simulink model "full_maneuver_platoon_new_strategy"  (R2019a)
settings: Solver=VariableStepAuto  StartTime=0.0  StopTime=70  FixedStep=0.1  MaxStep=0.05  RelTol=1e-3
libraries: simulink x97, dspsigops x7, powerlib_meascontrol x7, autolibshared x7
(part 5 of 7)

== system full_maneuver_platoon_new_strategy/Fo/Regular Vehicle Following/Velocity Control ==
  velocity : Inport
  realInput : Inport  Port=2
  intReset : Inport  Port=3
  Anti-windup gain : Gain  Gain=velKp/velKi
  Integrator2 : Integrator  ExternalReset=falling
  Sum : Sum  Inputs=|+-
  Sum1 : Sum  Inputs=|-+
  Sum2 : Sum  Inputs=-+|
  Sum3 : Sum  Inputs=|++
  freeFlowVel : Constant  Value=freeFlowVel
  velKi : Gain  Gain=velKi
  velKp : Gain  Gain=velKp
  u : Outport
  wires:
  Sum/1 -> velKi/1, velKp/1
  velKp/1 -> Sum3/2
  velKi/1 -> Sum2/2
  Integrator2/1 -> Sum3/1
  velocity/1 -> Sum/2
  freeFlowVel/1 -> Sum/1
  intReset/1 -> Integrator2/2
  Sum3/1 -> Sum1/2, u/1
  Anti-windup gain/1 -> Sum2/1
  realInput/1 -> Sum1/1
  Sum1/1 -> Anti-windup gain/1
  Sum2/1 -> Integrator2/1

== system full_maneuver_platoon_new_strategy/Fo/Vehicle Following During LC/Compute Errors ==
  xf : Inport
  vf : Inport  Port=2
  xl : Inport  Port=3
  vl : Inport  Port=4
  lcFlag : Inport  Port=5
  Compare To Constant : simulink/Logic and Bit Operations/Compare To Constant  relop=<=  const=0  OutDataTypeStr=boolean
  Demux : Demux  Outputs=2
  Demux1 : Demux  Outputs=2
  Gain3 : Gain  Gain=velFilterGain
  Integrator : Integrator  InitialCondition=[h d0]
  Integrator1 : Integrator  InitialCondition=vx0
  Multiply : Product
  Mux : Mux  Inputs=2
  Mux1 : Mux  Inputs=2
  Product : Product
  Saturation : Saturate  UpperLimit=maxAcceleration  LowerLimit=minAcceleration
  Sum : Sum  Inputs=-+|
  Sum1 : Sum  Inputs=++|
  Sum2 : Sum  Inputs=+-|
  Sum3 : Sum  Inputs=|++
  Sum4 : Sum  Inputs=-+|
  Sum5 : Sum  Inputs=|+-
  Sum6 : Sum  Inputs=+-|
  Sum7 : Sum  Inputs=|++
  Sum8 : Sum  Inputs=|+-
  Switch : Switch  Criteria=u2 > Threshold
  d0 : Constant  Value=d0
  d0Lc : Constant  Value=d0Lc
  h : Constant  Value=h
  hFilterGain : Gain  Gain=hFilterGain
  hLc : Constant  Value=hLc
  vLen : Constant  Value=lr+lf
  eh : Outport
  ev : Outport  Port=2
  "gap " : Outport  Port=3
  unsafeFlag : Outport  Port=4
  wires:
  Sum4/1 -> ev/1
  d0Lc/1 -> Mux1/2
  hFilterGain/1 -> Integrator/1
  Demux/1 -> Multiply/2
  xf/1 -> Sum1/2
  Sum/1 -> Sum2/1, "gap "/1, Sum6/1  "gap"
  Multiply/1 -> Sum3/1
  Demux1/2 -> Sum7/2
  hLc/1 -> Mux1/1
  vLen/1 -> Sum1/1
  Demux/2 -> Sum3/2
  Switch/1 -> Sum5/1
  Sum5/1 -> hFilterGain/1
  vf/1 -> Multiply/1, Product/1, Sum4/1
  Sum1/1 -> Sum/1  "x (front bumber)"
  Sum3/1 -> Sum2/2  "desired  gap"
  h/1 -> Mux/1
  Product/1 -> Sum7/1
  xl/1 -> Sum/2
  lcFlag/1 -> Switch/2
  Sum2/1 -> eh/1
  Compare To Constant/1 -> unsafeFlag/1
  Demux1/1 -> Product/2
  Integrator/1 -> Sum5/2, Demux/1
  d0/1 -> Mux/2
  Mux1/1 -> Switch/1
  Sum7/1 -> Sum6/2  "safe  gap"
  Mux/1 -> Switch/3, Demux1/1  "min safe gap"
  Sum6/1 -> Compare To Constant/1
  Saturation/1 -> Integrator1/1
  Gain3/1 -> Saturation/1
  Integrator1/1 -> Sum4/2, Sum8/2
  Sum8/1 -> Gain3/1
  vl/1 -> Sum8/1

== system full_maneuver_platoon_new_strategy/Fo/Vehicle Following During LC/Subsystem ==
  note: Condition for Lane Changing Vehicle
  note: Condition for Gap Generating Vehicle
  ego : Inport  OutDataTypeStr=Bus: vehStatesBus
  futureLeader : Inport  Port=2  OutDataTypeStr=Bus: vehStatesBus
  lcFlag : Inport  Port=3
  AND : Logic  IconShape=distinctive  AllPortsSameDT=off  OutDataTypeStr=boolean
  AND1 : Logic  IconShape=distinctive  AllPortsSameDT=off  OutDataTypeStr=boolean
  Abs : Abs
  Abs1 : Abs
  Bus Selector1 : BusSelector  OutputSignals=Y
  Bus Selector2 : BusSelector  OutputSignals=Y
  Compare To Constant : simulink/Logic and Bit Operations/Compare To Constant  relop=<=  const=1.8  OutDataTypeStr=boolean
  Compare To Constant1 : simulink/Logic and Bit Operations/Compare To Constant  relop=<=  const=0.5  OutDataTypeStr=boolean
  NOT : Logic  Operator=NOT  IconShape=distinctive  AllPortsSameDT=off  OutDataTypeStr=boolean
  OR : Logic  Operator=OR  IconShape=distinctive  AllPortsSameDT=off  OutDataTypeStr=boolean
  Scope : Scope  NumInputPorts=2
  Sum : Sum  Inputs=|+-
  Sum1 : Sum  Inputs=-+|
  lcDone : Outport
  wires:
  futureLeader/1 -> Bus Selector1/1
  Bus Selector1/1 -> Sum1/1, Sum/2  "<Y>"
  AND/1 -> Scope/1, OR/1
  Sum/1 -> Abs1/1
  Compare To Constant/1 -> AND/1
  lcFlag/1 -> AND1/1, NOT/1
  ego/1 -> Bus Selector2/1
  NOT/1 -> AND/2
  Sum1/1 -> Abs/1
  Compare To Constant1/1 -> AND1/2
  OR/1 -> lcDone/1
  AND1/1 -> Scope/2, OR/2
  Bus Selector2/1 -> Sum/1, Sum1/2  "<Y>"
  Abs/1 -> Compare To Constant1/1
  Abs1/1 -> Compare To Constant/1

== system full_maneuver_platoon_new_strategy/Fo/Vehicle Following During LC/Veh Following ==
  eh : Inport
  ev : Inport  Port=2
  realInput : Inport  Port=3
  intReset : Inport  Port=4
  Anti-windup gain : Gain  Gain=sqrt(Ki/Kd)
  Integrator : Integrator  ExternalReset=rising
  Kd : Gain  Gain=Kd
  Ki : Gain  Gain=Ki
  Kp : Gain  Gain=Kp
  Saturation1 : Saturate  UpperLimit=maxHeadwayError  LowerLimit=minHeadwayError
  Scope : Scope  NumInputPorts=4
  Sum : Sum  Inputs=|-+
  Sum1 : Sum  Inputs=+++
  Sum5 : Sum  Inputs=-+|
  u : Outport
  wires:
  intReset/1 -> Integrator/2
  Sum/1 -> Anti-windup gain/1
  realInput/1 -> Sum/1
  Sum1/1 -> Scope/4, u/1, Sum/2
  eh/1 -> Saturation1/1
  Saturation1/1 -> Ki/1, Kp/1
  Kd/1 -> Sum1/3, Scope/3
  Kp/1 -> Scope/2, Sum1/2
  Integrator/1 -> Scope/1, Sum1/1
  Sum5/1 -> Integrator/1
  Anti-windup gain/1 -> Sum5/1
  Ki/1 -> Sum5/2
  ev/1 -> Kd/1

== system full_maneuver_platoon_new_strategy/Fo/Vehicle Following During LC/Velocity Control ==
  velocity : Inport
  realInput : Inport  Port=2
  intReset : Inport  Port=3
  Anti-windup gain : Gain  Gain=velKp/velKi
  Integrator2 : Integrator  ExternalReset=falling
  Sum : Sum  Inputs=|+-
  Sum1 : Sum  Inputs=|-+
  Sum2 : Sum  Inputs=-+|
  Sum3 : Sum  Inputs=|++
  freeFlowVel : Constant  Value=freeFlowVel
  velKi : Gain  Gain=velKi
  velKp : Gain  Gain=velKp
  u : Outport
  wires:
  Sum2/1 -> Integrator2/1
  Sum1/1 -> Anti-windup gain/1
  realInput/1 -> Sum1/1
  Anti-windup gain/1 -> Sum2/1
  Sum3/1 -> u/1, Sum1/2
  intReset/1 -> Integrator2/2
  freeFlowVel/1 -> Sum/1
  velocity/1 -> Sum/2
  Integrator2/1 -> Sum3/1
  velKi/1 -> Sum2/2
  velKp/1 -> Sum3/2
  Sum/1 -> velKp/1, velKi/1

== system full_maneuver_platoon_new_strategy/Fo/Virtual Vehicle Following/Compute Errors ==
  xf : Inport
  vf : Inport  Port=2
  xl : Inport  Port=3
  vl : Inport  Port=4
  lcFlag : Inport  Port=5
  Compare To Constant : simulink/Logic and Bit Operations/Compare To Constant  relop=<=  const=0  OutDataTypeStr=boolean
  Demux : Demux  Outputs=2
  Demux1 : Demux  Outputs=2
  Gain3 : Gain  Gain=velFilterGain/10
  Integrator : Integrator  InitialCondition=[h d0]
  Integrator1 : Integrator  InitialCondition=vx0
  Multiply : Product
  Mux : Mux  Inputs=2
  Mux1 : Mux  Inputs=2
  Product : Product
  Saturation : Saturate  UpperLimit=maxAcceleration  LowerLimit=minAcceleration
  Sum : Sum  Inputs=-+|
  Sum1 : Sum  Inputs=++|
  Sum2 : Sum  Inputs=+-|
  Sum3 : Sum  Inputs=|++
  Sum4 : Sum  Inputs=-+|
  Sum5 : Sum  Inputs=|+-
  Sum6 : Sum  Inputs=+-|
  Sum7 : Sum  Inputs=|++
  Sum8 : Sum  Inputs=|+-
  Switch : Switch  Criteria=u2 > Threshold
  d0 : Constant  Value=d0
  d0Lc : Constant  Value=d0Lc
  h : Constant  Value=h
  hFilterGain : Gain  Gain=hFilterGain
  hLc : Constant  Value=hLc
  vLen : Constant  Value=lr+lf
  eh : Outport
  ev : Outport  Port=2
  "gap " : Outport  Port=3
  unsafeFlag : Outport  Port=4
  wires:
  Sum6/1 -> Compare To Constant/1
  Mux/1 -> Demux1/1, Switch/3  "min safe gap"
  Sum7/1 -> Sum6/2  "safe  gap"
  Mux1/1 -> Switch/1
  d0/1 -> Mux/2
  Integrator/1 -> Demux/1, Sum5/2
  Demux1/1 -> Product/2
  Compare To Constant/1 -> unsafeFlag/1
  Sum2/1 -> eh/1
  lcFlag/1 -> Switch/2
  xl/1 -> Sum/2
  Product/1 -> Sum7/1
  h/1 -> Mux/1
  Sum3/1 -> Sum2/2  "desired  gap"
  Sum1/1 -> Sum/1  "x (front bumber)"
  vf/1 -> Sum4/1, Product/1, Multiply/1
  Sum5/1 -> hFilterGain/1
  Switch/1 -> Sum5/1
  Demux/2 -> Sum3/2
  vLen/1 -> Sum1/1
  hLc/1 -> Mux1/1
  Demux1/2 -> Sum7/2
  Multiply/1 -> Sum3/1
  Sum/1 -> Sum6/1, "gap "/1, Sum2/1  "gap"
  xf/1 -> Sum1/2
  Demux/1 -> Multiply/2
  hFilterGain/1 -> Integrator/1
  d0Lc/1 -> Mux1/2
  Sum4/1 -> ev/1
  Integrator1/1 -> Sum4/2, Sum8/2
  Gain3/1 -> Saturation/1
  Sum8/1 -> Gain3/1
  Saturation/1 -> Integrator1/1
  vl/1 -> Sum8/1

== system full_maneuver_platoon_new_strategy/Fo/Virtual Vehicle Following/Subsystem ==
  ego : Inport  OutDataTypeStr=Bus: vehStatesBus
  virtualLeader : Inport  Port=2  OutDataTypeStr=Bus: vehStatesBus
  Abs : Abs
  Bus Selector : BusSelector  OutputSignals=Y
  Bus Selector1 : BusSelector  OutputSignals=Y
  Compare To Constant : simulink/Logic and Bit Operations/Compare To Constant  relop=<  const=3.6-0.5  OutDataTypeStr=boolean
  Scope : Scope  NumInputPorts=3
  Sum : Sum  Inputs=+-
  lcStarted : Outport
  wires:
  ego/1 -> Bus Selector/1
  virtualLeader/1 -> Bus Selector1/1
  Bus Selector/1 -> Scope/1, Sum/1  "<Y>"
  Bus Selector1/1 -> Sum/2, Scope/2  "<Y>"
  Compare To Constant/1 -> lcStarted/1
  Sum/1 -> Abs/1
  Abs/1 -> Scope/3, Compare To Constant/1

== system full_maneuver_platoon_new_strategy/Fo/Virtual Vehicle Following/Velocity Control ==
  note: Velocity control
  intReset : Inport
  ev : Inport  Port=2
  Integrator2 : Integrator  ExternalReset=rising
  Sum3 : Sum
  velKi : Gain  Gain=velKi
  velKp : Gain  Gain=velKp
  Out1 : Outport
  wires:
  Integrator2/1 -> velKi/1
  velKi/1 -> Sum3/2
  Sum3/1 -> Out1/1
  velKp/1 -> Sum3/1
  ev/1 -> velKp/1, Integrator2/1
  intReset/1 -> Integrator2/2

== system full_maneuver_platoon_new_strategy/Fo/Virtual Vehicle Following/Virtual Leader Following ==
  eh : Inport
  ev : Inport  Port=2
  realInput : Inport  Port=3
  Anti-windup gain : Gain  Gain=sqrt(Ki/Kd)
  Integrator : Integrator
  Kd : Gain  Gain=Kd
  Ki : Gain  Gain=Ki
  Kp : Gain  Gain=Kp
  Saturation1 : Saturate  UpperLimit=maxHeadwayError  LowerLimit=minHeadwayError
  Scope : Scope  NumInputPorts=3
  Sum : Sum  Inputs=|-+
  Sum1 : Sum  Inputs=+++
  Sum5 : Sum  Inputs=-+|
  u : Outport
  wires:
  ev/1 -> Kd/1
  Ki/1 -> Sum5/2
  Anti-windup gain/1 -> Sum5/1
  Sum5/1 -> Integrator/1
  Integrator/1 -> Scope/1, Sum1/1
  Kp/1 -> Scope/2, Sum1/2
  Kd/1 -> Scope/3, Sum1/3
  Saturation1/1 -> Kp/1, Ki/1
  eh/1 -> Saturation1/1
  Sum1/1 -> Sum/2, u/1
  realInput/1 -> Sum/1
  Sum/1 -> Anti-windup gain/1

== system full_maneuver_platoon_new_strategy/Fo/followerErrors/gapToFollower ==
  xf : Inport
  vf : Inport  Port=2
  xl : Inport  Port=3
  Multiply : Product
  Sum : Sum  Inputs=-+|
  Sum1 : Sum  Inputs=++|
  Sum2 : Sum  Inputs=+-|
  Sum3 : Sum  Inputs=|++
  d0 : Constant  Value=d0
  h : Constant  Value=h
  vLen : Constant  Value=lr+lf
  eh : Outport
  "gap " : Outport  Port=2
  wires:
  vLen/1 -> Sum1/1
  Multiply/1 -> Sum3/1
  Sum/1 -> "gap "/1, Sum2/1  "gap"
  xf/1 -> Sum1/2
  Sum3/1 -> Sum2/2  "desired  gap"
  vf/1 -> Multiply/1
  Sum1/1 -> Sum/1  "x (front bumber)"
  xl/1 -> Sum/2
  Sum2/1 -> eh/1
  h/1 -> Multiply/2  "time headway"
  d0/1 -> Sum3/2  "gap at  standstill"

== system full_maneuver_platoon_new_strategy/Ld/Lateral Control/Full State Observer ==
  note: yhat
  note: xhat
  measuredOutputs : Inport
  delta : Inport  Port=2
  Add1 : Sum  Inputs=|-+
  Gain : Gain  Gain=B  Multiplication=Matrix(K*u)
  Gain1 : Gain  Gain=C  Multiplication=Matrix(K*u)
  Gain2 : Gain  Gain=L  Multiplication=Matrix(K*u)
  Gain3 : Gain  Gain=A  Multiplication=Matrix(K*u)
  Integrator : Integrator  InitialCondition=[y0; 0; 0; 0]
  Signal Specification : SignalSpecification  Dimensions=[size(C,1) 1]
  Sum : Sum  Inputs=+++
  xhat : Outport
  wires:
  Gain2/1 -> Sum/1
  Signal Specification/1 -> Gain2/1
  Gain3/1 -> Sum/2
  Gain/1 -> Sum/3
  delta/1 -> Gain/1
  measuredOutputs/1 -> Add1/2
  Sum/1 -> Integrator/1
  Gain1/1 -> Add1/1
  Integrator/1 -> Gain1/1, Gain3/1, xhat/1
  Add1/1 -> Signal Specification/1

== system full_maneuver_platoon_new_strategy/Ld/Lateral Control/Triggered Subsystem1 ==
  In1 : Inport
  Trigger : TriggerPort  VariantControl=Variant
  Out1 : Outport  InitialOutput=y0
  wires:
  In1/1 -> Out1/1

== system full_maneuver_platoon_new_strategy/Ld/Regular Vehicle Following/Compute Errors ==
  xf : Inport
  vf : Inport  Port=2
  xl : Inport  Port=3
  vl : Inport  Port=4
  lcFlag : Inport  Port=5
  Compare To Constant : simulink/Logic and Bit Operations/Compare To Constant  relop=<=  const=0  OutDataTypeStr=boolean
  Demux : Demux  Outputs=2
  Demux1 : Demux  Outputs=2
  Gain3 : Gain  Gain=velFilterGain
  Integrator : Integrator  InitialCondition=[h d0]
  Integrator1 : Integrator  InitialCondition=vx0
  Multiply : Product
  Mux : Mux  Inputs=2
  Mux1 : Mux  Inputs=2
  Product : Product
  Saturation : Saturate  UpperLimit=maxAcceleration  LowerLimit=minAcceleration
  Sum : Sum  Inputs=-+|
  Sum1 : Sum  Inputs=++|
  Sum2 : Sum  Inputs=+-|
  Sum3 : Sum  Inputs=|++
  Sum4 : Sum  Inputs=-+|
  Sum5 : Sum  Inputs=|+-
  Sum6 : Sum  Inputs=+-|
  Sum7 : Sum  Inputs=|++
  Sum8 : Sum  Inputs=|+-
  Switch : Switch  Criteria=u2 > Threshold
  d0 : Constant  Value=d0
  d0Lc : Constant  Value=d0Lc
  h : Constant  Value=h
  hFilterGain : Gain  Gain=hFilterGain
  hLc : Constant  Value=hLc
  vLen : Constant  Value=lr+lf
  eh : Outport
  ev : Outport  Port=2
  "gap " : Outport  Port=3
  unsafeFlag : Outport  Port=4
  wires:
  Sum6/1 -> Compare To Constant/1
  Mux/1 -> Demux1/1, Switch/3  "min safe gap"
  Sum7/1 -> Sum6/2  "safe  gap"
  Mux1/1 -> Switch/1
  d0/1 -> Mux/2
  Integrator/1 -> Demux/1, Sum5/2
  Demux1/1 -> Product/2
  Compare To Constant/1 -> unsafeFlag/1
  Sum2/1 -> eh/1
  lcFlag/1 -> Switch/2
  xl/1 -> Sum/2
  Product/1 -> Sum7/1
  h/1 -> Mux/1
  Sum3/1 -> Sum2/2  "desired  gap"
  Sum1/1 -> Sum/1  "x (front bumber)"
  vf/1 -> Sum4/1, Product/1, Multiply/1
  Sum5/1 -> hFilterGain/1
  Switch/1 -> Sum5/1
  Demux/2 -> Sum3/2
  vLen/1 -> Sum1/1
  hLc/1 -> Mux1/1
  Demux1/2 -> Sum7/2
  Multiply/1 -> Sum3/1
  Sum/1 -> Sum6/1, "gap "/1, Sum2/1  "gap"
  xf/1 -> Sum1/2
  Demux/1 -> Multiply/2
  hFilterGain/1 -> Integrator/1
  d0Lc/1 -> Mux1/2
  vl/1 -> Sum8/1
  Sum4/1 -> ev/1
  Gain3/1 -> Saturation/1
  Saturation/1 -> Integrator1/1
  Integrator1/1 -> Sum4/2, Sum8/2
  Sum8/1 -> Gain3/1

== system full_maneuver_platoon_new_strategy/Ld/Regular Vehicle Following/Veh Following ==
  eh : Inport
  ev : Inport  Port=2
  realInput : Inport  Port=3
  intReset : Inport  Port=4
  Anti-windup gain : Gain  Gain=sqrt(Ki/Kd)
  Integrator : Integrator  ExternalReset=rising
  Kd : Gain  Gain=Kd
  Ki : Gain  Gain=Ki
  Kp : Gain  Gain=Kp
  Saturation1 : Saturate  UpperLimit=maxHeadwayError  LowerLimit=minHeadwayError
  Scope : Scope  NumInputPorts=4
  Sum : Sum  Inputs=|-+
  Sum1 : Sum  Inputs=+++
  Sum5 : Sum  Inputs=-+|
  u : Outport
  wires:
  ev/1 -> Kd/1
  Ki/1 -> Sum5/2
  Anti-windup gain/1 -> Sum5/1
  Sum5/1 -> Integrator/1
  Integrator/1 -> Sum1/1, Scope/1
  Kp/1 -> Sum1/2, Scope/2
  Kd/1 -> Scope/3, Sum1/3
  Saturation1/1 -> Kp/1, Ki/1
  eh/1 -> Saturation1/1
  Sum1/1 -> Sum/2, u/1, Scope/4
  realInput/1 -> Sum/1
  Sum/1 -> Anti-windup gain/1
  intReset/1 -> Integrator/2

== system full_maneuver_platoon_new_strategy/Ld/Regular Vehicle Following/Velocity Control ==
  velocity : Inport
  realInput : Inport  Port=2
  intReset : Inport  Port=3
  Anti-windup gain : Gain  Gain=velKp/velKi
  Integrator2 : Integrator  ExternalReset=falling
  Sum : Sum  Inputs=|+-
  Sum1 : Sum  Inputs=|-+
  Sum2 : Sum  Inputs=-+|
  Sum3 : Sum  Inputs=|++
  freeFlowVel : Constant  Value=freeFlowVel
  velKi : Gain  Gain=velKi
  velKp : Gain  Gain=velKp
  u : Outport
  wires:
  Sum/1 -> velKi/1, velKp/1
  velKp/1 -> Sum3/2
  velKi/1 -> Sum2/2
  Integrator2/1 -> Sum3/1
  velocity/1 -> Sum/2
  freeFlowVel/1 -> Sum/1
  intReset/1 -> Integrator2/2
  Sum3/1 -> Sum1/2, u/1
  Anti-windup gain/1 -> Sum2/1
  realInput/1 -> Sum1/1
  Sum1/1 -> Anti-windup gain/1
  Sum2/1 -> Integrator2/1

== system full_maneuver_platoon_new_strategy/Ld/Vehicle Following During LC/Compute Errors ==
  xf : Inport
  vf : Inport  Port=2
  xl : Inport  Port=3
  vl : Inport  Port=4
  lcFlag : Inport  Port=5
  Compare To Constant : simulink/Logic and Bit Operations/Compare To Constant  relop=<=  const=0  OutDataTypeStr=boolean
  Demux : Demux  Outputs=2
  Demux1 : Demux  Outputs=2
  Gain3 : Gain  Gain=velFilterGain
  Integrator : Integrator  InitialCondition=[h d0]
  Integrator1 : Integrator  InitialCondition=vx0
  Multiply : Product
  Mux : Mux  Inputs=2
  Mux1 : Mux  Inputs=2
  Product : Product
  Saturation : Saturate  UpperLimit=maxAcceleration  LowerLimit=minAcceleration
  Sum : Sum  Inputs=-+|
  Sum1 : Sum  Inputs=++|
  Sum2 : Sum  Inputs=+-|
  Sum3 : Sum  Inputs=|++
  Sum4 : Sum  Inputs=-+|
  Sum5 : Sum  Inputs=|+-
  Sum6 : Sum  Inputs=+-|
  Sum7 : Sum  Inputs=|++
  Sum8 : Sum  Inputs=|+-
  Switch : Switch  Criteria=u2 > Threshold
  d0 : Constant  Value=d0
  d0Lc : Constant  Value=d0Lc
  h : Constant  Value=h
  hFilterGain : Gain  Gain=hFilterGain
  hLc : Constant  Value=hLc
  vLen : Constant  Value=lr+lf
  eh : Outport
  ev : Outport  Port=2
  "gap " : Outport  Port=3
  unsafeFlag : Outport  Port=4
  wires:
  Sum4/1 -> ev/1
  d0Lc/1 -> Mux1/2
  hFilterGain/1 -> Integrator/1
  Demux/1 -> Multiply/2
  xf/1 -> Sum1/2
  Sum/1 -> Sum2/1, "gap "/1, Sum6/1  "gap"
  Multiply/1 -> Sum3/1
  Demux1/2 -> Sum7/2
  hLc/1 -> Mux1/1
  vLen/1 -> Sum1/1
  Demux/2 -> Sum3/2
  Switch/1 -> Sum5/1
  Sum5/1 -> hFilterGain/1
  vf/1 -> Multiply/1, Product/1, Sum4/1
  Sum1/1 -> Sum/1  "x (front bumber)"
  Sum3/1 -> Sum2/2  "desired  gap"
  h/1 -> Mux/1
  Product/1 -> Sum7/1
  xl/1 -> Sum/2
  lcFlag/1 -> Switch/2
  Sum2/1 -> eh/1
  Compare To Constant/1 -> unsafeFlag/1
  Demux1/1 -> Product/2
  Integrator/1 -> Sum5/2, Demux/1
  d0/1 -> Mux/2
  Mux1/1 -> Switch/1
  Sum7/1 -> Sum6/2  "safe  gap"
  Mux/1 -> Switch/3, Demux1/1  "min safe gap"
  Sum6/1 -> Compare To Constant/1
  Saturation/1 -> Integrator1/1
  Gain3/1 -> Saturation/1
  Integrator1/1 -> Sum4/2, Sum8/2
  Sum8/1 -> Gain3/1
  vl/1 -> Sum8/1

== system full_maneuver_platoon_new_strategy/Ld/Vehicle Following During LC/Subsystem ==
  note: Condition for Lane Changing Vehicle
  note: Condition for Gap Generating Vehicle
  ego : Inport  OutDataTypeStr=Bus: vehStatesBus
  futureLeader : Inport  Port=2  OutDataTypeStr=Bus: vehStatesBus
  lcFlag : Inport  Port=3
  AND : Logic  IconShape=distinctive  AllPortsSameDT=off  OutDataTypeStr=boolean
  AND1 : Logic  IconShape=distinctive  AllPortsSameDT=off  OutDataTypeStr=boolean
  Abs : Abs
  Abs1 : Abs
  Bus Selector1 : BusSelector  OutputSignals=Y
  Bus Selector2 : BusSelector  OutputSignals=Y
  Compare To Constant : simulink/Logic and Bit Operations/Compare To Constant  relop=<=  const=1.8  OutDataTypeStr=boolean
  Compare To Constant1 : simulink/Logic and Bit Operations/Compare To Constant  relop=<=  const=0.5  OutDataTypeStr=boolean
  NOT : Logic  Operator=NOT  IconShape=distinctive  AllPortsSameDT=off  OutDataTypeStr=boolean
  OR : Logic  Operator=OR  IconShape=distinctive  AllPortsSameDT=off  OutDataTypeStr=boolean
  Scope : Scope  NumInputPorts=2
  Sum : Sum  Inputs=|+-
  Sum1 : Sum  Inputs=-+|
  lcDone : Outport
  wires:
  futureLeader/1 -> Bus Selector1/1
  Bus Selector1/1 -> Sum1/1, Sum/2  "<Y>"
  AND/1 -> Scope/1, OR/1
  Sum/1 -> Abs1/1
  Compare To Constant/1 -> AND/1
  lcFlag/1 -> AND1/1, NOT/1
  ego/1 -> Bus Selector2/1
  NOT/1 -> AND/2
  Sum1/1 -> Abs/1
  Compare To Constant1/1 -> AND1/2
  OR/1 -> lcDone/1
  AND1/1 -> Scope/2, OR/2
  Bus Selector2/1 -> Sum/1, Sum1/2  "<Y>"
  Abs/1 -> Compare To Constant1/1
  Abs1/1 -> Compare To Constant/1

== system full_maneuver_platoon_new_strategy/Ld/Vehicle Following During LC/Veh Following ==
  eh : Inport
  ev : Inport  Port=2
  realInput : Inport  Port=3
  intReset : Inport  Port=4
  Anti-windup gain : Gain  Gain=sqrt(Ki/Kd)
  Integrator : Integrator  ExternalReset=rising
  Kd : Gain  Gain=Kd
  Ki : Gain  Gain=Ki
  Kp : Gain  Gain=Kp
  Saturation1 : Saturate  UpperLimit=maxHeadwayError  LowerLimit=minHeadwayError
  Scope : Scope  NumInputPorts=4
  Sum : Sum  Inputs=|-+
  Sum1 : Sum  Inputs=+++
  Sum5 : Sum  Inputs=-+|
  u : Outport
  wires:
  intReset/1 -> Integrator/2
  Sum/1 -> Anti-windup gain/1
  realInput/1 -> Sum/1
  Sum1/1 -> Scope/4, u/1, Sum/2
  eh/1 -> Saturation1/1
  Saturation1/1 -> Ki/1, Kp/1
  Kd/1 -> Sum1/3, Scope/3
  Kp/1 -> Scope/2, Sum1/2
  Integrator/1 -> Scope/1, Sum1/1
  Sum5/1 -> Integrator/1
  Anti-windup gain/1 -> Sum5/1
  Ki/1 -> Sum5/2
  ev/1 -> Kd/1

== system full_maneuver_platoon_new_strategy/Ld/Vehicle Following During LC/Velocity Control ==
  velocity : Inport
  realInput : Inport  Port=2
  intReset : Inport  Port=3
  Anti-windup gain : Gain  Gain=velKp/velKi
  Integrator2 : Integrator  ExternalReset=falling
  Sum : Sum  Inputs=|+-
  Sum1 : Sum  Inputs=|-+
  Sum2 : Sum  Inputs=-+|
  Sum3 : Sum  Inputs=|++
  freeFlowVel : Constant  Value=freeFlowVel
  velKi : Gain  Gain=velKi
  velKp : Gain  Gain=velKp
  u : Outport
  wires:
  Sum2/1 -> Integrator2/1
  Sum1/1 -> Anti-windup gain/1
  realInput/1 -> Sum1/1
  Anti-windup gain/1 -> Sum2/1
  Sum3/1 -> u/1, Sum1/2
  intReset/1 -> Integrator2/2
  freeFlowVel/1 -> Sum/1
  velocity/1 -> Sum/2
  Integrator2/1 -> Sum3/1
  velKi/1 -> Sum2/2
  velKp/1 -> Sum3/2
  Sum/1 -> velKp/1, velKi/1

== system full_maneuver_platoon_new_strategy/Ld/Virtual Vehicle Following/Compute Errors ==
  xf : Inport
  vf : Inport  Port=2
  xl : Inport  Port=3
  vl : Inport  Port=4
  lcFlag : Inport  Port=5
  Compare To Constant : simulink/Logic and Bit Operations/Compare To Constant  relop=<=  const=0  OutDataTypeStr=boolean
  Demux : Demux  Outputs=2
  Demux1 : Demux  Outputs=2
  Gain3 : Gain  Gain=velFilterGain/10
  Integrator : Integrator  InitialCondition=[h d0]
  Integrator1 : Integrator  InitialCondition=vx0
  Multiply : Product
  Mux : Mux  Inputs=2
  Mux1 : Mux  Inputs=2
  Product : Product
  Saturation : Saturate  UpperLimit=maxAcceleration  LowerLimit=minAcceleration
  Sum : Sum  Inputs=-+|
  Sum1 : Sum  Inputs=++|
  Sum2 : Sum  Inputs=+-|
  Sum3 : Sum  Inputs=|++
  Sum4 : Sum  Inputs=-+|
  Sum5 : Sum  Inputs=|+-
  Sum6 : Sum  Inputs=+-|
  Sum7 : Sum  Inputs=|++
  Sum8 : Sum  Inputs=|+-
  Switch : Switch  Criteria=u2 > Threshold
  d0 : Constant  Value=d0
  d0Lc : Constant  Value=d0Lc
  h : Constant  Value=h
  hFilterGain : Gain  Gain=hFilterGain
  hLc : Constant  Value=hLc
  vLen : Constant  Value=lr+lf
  eh : Outport
  ev : Outport  Port=2
  "gap " : Outport  Port=3
  unsafeFlag : Outport  Port=4
  wires:
  Sum6/1 -> Compare To Constant/1
  Mux/1 -> Demux1/1, Switch/3  "min safe gap"
  Sum7/1 -> Sum6/2  "safe  gap"
  Mux1/1 -> Switch/1
  d0/1 -> Mux/2
  Integrator/1 -> Demux/1, Sum5/2
  Demux1/1 -> Product/2
  Compare To Constant/1 -> unsafeFlag/1
  Sum2/1 -> eh/1
  lcFlag/1 -> Switch/2
  xl/1 -> Sum/2
  Product/1 -> Sum7/1
  h/1 -> Mux/1
  Sum3/1 -> Sum2/2  "desired  gap"
  Sum1/1 -> Sum/1  "x (front bumber)"
  vf/1 -> Sum4/1, Product/1, Multiply/1
  Sum5/1 -> hFilterGain/1
  Switch/1 -> Sum5/1
  Demux/2 -> Sum3/2
  vLen/1 -> Sum1/1
  hLc/1 -> Mux1/1
  Demux1/2 -> Sum7/2
  Multiply/1 -> Sum3/1
  Sum/1 -> Sum6/1, "gap "/1, Sum2/1  "gap"
  xf/1 -> Sum1/2
  Demux/1 -> Multiply/2
  hFilterGain/1 -> Integrator/1
  d0Lc/1 -> Mux1/2
  Sum4/1 -> ev/1
  Integrator1/1 -> Sum4/2, Sum8/2
  Gain3/1 -> Saturation/1
  Sum8/1 -> Gain3/1
  Saturation/1 -> Integrator1/1
  vl/1 -> Sum8/1

== system full_maneuver_platoon_new_strategy/Ld/Virtual Vehicle Following/Subsystem ==
  ego : Inport  OutDataTypeStr=Bus: vehStatesBus
  virtualLeader : Inport  Port=2  OutDataTypeStr=Bus: vehStatesBus
  Abs : Abs
  Bus Selector : BusSelector  OutputSignals=Y
  Bus Selector1 : BusSelector  OutputSignals=Y
  Compare To Constant : simulink/Logic and Bit Operations/Compare To Constant  relop=<  const=3.6-0.5  OutDataTypeStr=boolean
  Scope : Scope  NumInputPorts=3
  Sum : Sum  Inputs=+-
  lcStarted : Outport
  wires:
  ego/1 -> Bus Selector/1
  virtualLeader/1 -> Bus Selector1/1
  Bus Selector/1 -> Scope/1, Sum/1  "<Y>"
  Bus Selector1/1 -> Sum/2, Scope/2  "<Y>"
  Compare To Constant/1 -> lcStarted/1
  Sum/1 -> Abs/1
  Abs/1 -> Scope/3, Compare To Constant/1

== system full_maneuver_platoon_new_strategy/Ld/Virtual Vehicle Following/Velocity Control ==
  note: Velocity control
  intReset : Inport
  ev : Inport  Port=2
  Integrator2 : Integrator  ExternalReset=rising
  Sum3 : Sum
  velKi : Gain  Gain=velKi
  velKp : Gain  Gain=velKp
  Out1 : Outport
  wires:
  Integrator2/1 -> velKi/1
  velKi/1 -> Sum3/2
  Sum3/1 -> Out1/1
  velKp/1 -> Sum3/1
  ev/1 -> velKp/1, Integrator2/1
  intReset/1 -> Integrator2/2

== system full_maneuver_platoon_new_strategy/Ld/Virtual Vehicle Following/Virtual Leader Following ==
  eh : Inport
  ev : Inport  Port=2
  realInput : Inport  Port=3
  Anti-windup gain : Gain  Gain=sqrt(Ki/Kd)
  Integrator : Integrator
  Kd : Gain  Gain=Kd
  Ki : Gain  Gain=Ki
  Kp : Gain  Gain=Kp
  Saturation1 : Saturate  UpperLimit=maxHeadwayError  LowerLimit=minHeadwayError
  Scope : Scope  NumInputPorts=3
  Sum : Sum  Inputs=|-+
  Sum1 : Sum  Inputs=+++
  Sum5 : Sum  Inputs=-+|
  u : Outport
  wires:
  ev/1 -> Kd/1
  Ki/1 -> Sum5/2
  Anti-windup gain/1 -> Sum5/1
  Sum5/1 -> Integrator/1
  Integrator/1 -> Scope/1, Sum1/1
  Kp/1 -> Scope/2, Sum1/2
  Kd/1 -> Scope/3, Sum1/3
  Saturation1/1 -> Kp/1, Ki/1
  eh/1 -> Saturation1/1
  Sum1/1 -> Sum/2, u/1
  realInput/1 -> Sum/1
  Sum/1 -> Anti-windup gain/1

== system full_maneuver_platoon_new_strategy/Ld/followerErrors/gapToFollower ==
  xf : Inport
  vf : Inport  Port=2
  xl : Inport  Port=3
  Multiply : Product
  Sum : Sum  Inputs=-+|
  Sum1 : Sum  Inputs=++|
  Sum2 : Sum  Inputs=+-|
  Sum3 : Sum  Inputs=|++
  d0 : Constant  Value=d0
  h : Constant  Value=h
  vLen : Constant  Value=lr+lf
  eh : Outport
  "gap " : Outport  Port=2
  wires:
  vLen/1 -> Sum1/1
  Multiply/1 -> Sum3/1
  Sum/1 -> "gap "/1, Sum2/1  "gap"
  xf/1 -> Sum1/2
  Sum3/1 -> Sum2/2  "desired  gap"
  vf/1 -> Multiply/1
  Sum1/1 -> Sum/1  "x (front bumber)"
  xl/1 -> Sum/2
  Sum2/1 -> eh/1
  h/1 -> Multiply/2  "time headway"
  d0/1 -> Sum3/2  "gap at  standstill"

== system full_maneuver_platoon_new_strategy/Lo/Lateral Control/Full State Observer ==
  note: xhat
  note: yhat
  measuredOutputs : Inport
  delta : Inport  Port=2
  Add1 : Sum  Inputs=|-+
  Gain : Gain  Gain=B  Multiplication=Matrix(K*u)
  Gain1 : Gain  Gain=C  Multiplication=Matrix(K*u)
  Gain2 : Gain  Gain=L  Multiplication=Matrix(K*u)
  Gain3 : Gain  Gain=A  Multiplication=Matrix(K*u)
  Integrator : Integrator  InitialCondition=[y0; 0; 0; 0]
  Signal Specification : SignalSpecification  Dimensions=[size(C,1) 1]
  Sum : Sum  Inputs=+++
  xhat : Outport
  wires:
  Add1/1 -> Signal Specification/1
  Integrator/1 -> xhat/1, Gain3/1, Gain1/1
  Gain1/1 -> Add1/1
  Sum/1 -> Integrator/1
  measuredOutputs/1 -> Add1/2
  delta/1 -> Gain/1
  Gain/1 -> Sum/3
  Gain3/1 -> Sum/2
  Signal Specification/1 -> Gain2/1
  Gain2/1 -> Sum/1

== system full_maneuver_platoon_new_strategy/Lo/Lateral Control/Triggered Subsystem1 ==
  In1 : Inport
  Trigger : TriggerPort  VariantControl=Variant
  Out1 : Outport  InitialOutput=y0
  wires:
  In1/1 -> Out1/1

== system full_maneuver_platoon_new_strategy/Lo/Regular Vehicle Following/Compute Errors ==
  xf : Inport
  vf : Inport  Port=2
  xl : Inport  Port=3
  vl : Inport  Port=4
  lcFlag : Inport  Port=5
  Compare To Constant : simulink/Logic and Bit Operations/Compare To Constant  relop=<=  const=0  OutDataTypeStr=boolean
  Demux : Demux  Outputs=2
  Demux1 : Demux  Outputs=2
  Gain3 : Gain  Gain=velFilterGain
  Integrator : Integrator  InitialCondition=[h d0]
  Integrator1 : Integrator  InitialCondition=vx0
  Multiply : Product
  Mux : Mux  Inputs=2
  Mux1 : Mux  Inputs=2
  Product : Product
  Saturation : Saturate  UpperLimit=maxAcceleration  LowerLimit=minAcceleration
  Sum : Sum  Inputs=-+|
  Sum1 : Sum  Inputs=++|
  Sum2 : Sum  Inputs=+-|
  Sum3 : Sum  Inputs=|++
  Sum4 : Sum  Inputs=-+|
  Sum5 : Sum  Inputs=|+-
  Sum6 : Sum  Inputs=+-|
  Sum7 : Sum  Inputs=|++
  Sum8 : Sum  Inputs=|+-
  Switch : Switch  Criteria=u2 > Threshold
  d0 : Constant  Value=d0
  d0Lc : Constant  Value=d0Lc
  h : Constant  Value=h
  hFilterGain : Gain  Gain=hFilterGain
  hLc : Constant  Value=hLc
  vLen : Constant  Value=lr+lf
  eh : Outport
  ev : Outport  Port=2
  "gap " : Outport  Port=3
  unsafeFlag : Outport  Port=4
  wires:
  Sum8/1 -> Gain3/1
  Integrator1/1 -> Sum8/2, Sum4/2
  Saturation/1 -> Integrator1/1
  Gain3/1 -> Saturation/1
  Sum4/1 -> ev/1
  vl/1 -> Sum8/1
  d0Lc/1 -> Mux1/2
  hFilterGain/1 -> Integrator/1
  Demux/1 -> Multiply/2
  xf/1 -> Sum1/2
  Sum/1 -> Sum2/1, "gap "/1, Sum6/1  "gap"
  Multiply/1 -> Sum3/1
  Demux1/2 -> Sum7/2
  hLc/1 -> Mux1/1
  vLen/1 -> Sum1/1
  Demux/2 -> Sum3/2
  Switch/1 -> Sum5/1
  Sum5/1 -> hFilterGain/1
  vf/1 -> Multiply/1, Product/1, Sum4/1
  Sum1/1 -> Sum/1  "x (front bumber)"
  Sum3/1 -> Sum2/2  "desired  gap"
  h/1 -> Mux/1
  Product/1 -> Sum7/1
  xl/1 -> Sum/2
  lcFlag/1 -> Switch/2
  Sum2/1 -> eh/1
  Compare To Constant/1 -> unsafeFlag/1
  Demux1/1 -> Product/2
  Integrator/1 -> Sum5/2, Demux/1
  d0/1 -> Mux/2
  Mux1/1 -> Switch/1
  Sum7/1 -> Sum6/2  "safe  gap"
  Mux/1 -> Switch/3, Demux1/1  "min safe gap"
  Sum6/1 -> Compare To Constant/1

== system full_maneuver_platoon_new_strategy/Lo/Regular Vehicle Following/Veh Following ==
  eh : Inport
  ev : Inport  Port=2
  realInput : Inport  Port=3
  intReset : Inport  Port=4
  Anti-windup gain : Gain  Gain=sqrt(Ki/Kd)
  Integrator : Integrator  ExternalReset=rising
  Kd : Gain  Gain=Kd
  Ki : Gain  Gain=Ki
  Kp : Gain  Gain=Kp
  Saturation1 : Saturate  UpperLimit=maxHeadwayError  LowerLimit=minHeadwayError
  Scope : Scope  NumInputPorts=4
  Sum : Sum  Inputs=|-+
  Sum1 : Sum  Inputs=+++
  Sum5 : Sum  Inputs=-+|
  u : Outport
  wires:
  intReset/1 -> Integrator/2
  Sum/1 -> Anti-windup gain/1
  realInput/1 -> Sum/1
  Sum1/1 -> Scope/4, u/1, Sum/2
  eh/1 -> Saturation1/1
  Saturation1/1 -> Ki/1, Kp/1
  Kd/1 -> Sum1/3, Scope/3
  Kp/1 -> Scope/2, Sum1/2
  Integrator/1 -> Scope/1, Sum1/1
  Sum5/1 -> Integrator/1
  Anti-windup gain/1 -> Sum5/1
  Ki/1 -> Sum5/2
  ev/1 -> Kd/1

== system full_maneuver_platoon_new_strategy/Lo/Regular Vehicle Following/Velocity Control ==
  velocity : Inport
  realInput : Inport  Port=2
  intReset : Inport  Port=3
  Anti-windup gain : Gain  Gain=velKp/velKi
  Integrator2 : Integrator  ExternalReset=falling
  Sum : Sum  Inputs=|+-
  Sum1 : Sum  Inputs=|-+
  Sum2 : Sum  Inputs=-+|
  Sum3 : Sum  Inputs=|++
  freeFlowVel : Constant  Value=freeFlowVel
  velKi : Gain  Gain=velKi
  velKp : Gain  Gain=velKp
  u : Outport
  wires:
  Sum2/1 -> Integrator2/1
  Sum1/1 -> Anti-windup gain/1
  realInput/1 -> Sum1/1
  Anti-windup gain/1 -> Sum2/1
  Sum3/1 -> u/1, Sum1/2
  intReset/1 -> Integrator2/2
  freeFlowVel/1 -> Sum/1
  velocity/1 -> Sum/2
  Integrator2/1 -> Sum3/1
  velKi/1 -> Sum2/2
  velKp/1 -> Sum3/2
  Sum/1 -> velKp/1, velKi/1

== system full_maneuver_platoon_new_strategy/Lo/Vehicle Following During LC/Compute Errors ==
  xf : Inport
  vf : Inport  Port=2
  xl : Inport  Port=3
  vl : Inport  Port=4
  lcFlag : Inport  Port=5
  Compare To Constant : simulink/Logic and Bit Operations/Compare To Constant  relop=<=  const=0  OutDataTypeStr=boolean
  Demux : Demux  Outputs=2
  Demux1 : Demux  Outputs=2
  Gain3 : Gain  Gain=velFilterGain
  Integrator : Integrator  InitialCondition=[h d0]
  Integrator1 : Integrator  InitialCondition=vx0
  Multiply : Product
  Mux : Mux  Inputs=2
  Mux1 : Mux  Inputs=2
  Product : Product
  Saturation : Saturate  UpperLimit=maxAcceleration  LowerLimit=minAcceleration
  Sum : Sum  Inputs=-+|
  Sum1 : Sum  Inputs=++|
  Sum2 : Sum  Inputs=+-|
  Sum3 : Sum  Inputs=|++
  Sum4 : Sum  Inputs=-+|
  Sum5 : Sum  Inputs=|+-
  Sum6 : Sum  Inputs=+-|
  Sum7 : Sum  Inputs=|++
  Sum8 : Sum  Inputs=|+-
  Switch : Switch  Criteria=u2 > Threshold
  d0 : Constant  Value=d0
  d0Lc : Constant  Value=d0Lc
  h : Constant  Value=h
  hFilterGain : Gain  Gain=hFilterGain
  hLc : Constant  Value=hLc
  vLen : Constant  Value=lr+lf
  eh : Outport
  ev : Outport  Port=2
  "gap " : Outport  Port=3
  unsafeFlag : Outport  Port=4
  wires:
  vl/1 -> Sum8/1
  Sum8/1 -> Gain3/1
  Integrator1/1 -> Sum8/2, Sum4/2
  Gain3/1 -> Saturation/1
  Saturation/1 -> Integrator1/1
  Sum6/1 -> Compare To Constant/1
  Mux/1 -> Demux1/1, Switch/3  "min safe gap"
  Sum7/1 -> Sum6/2  "safe  gap"
  Mux1/1 -> Switch/1
  d0/1 -> Mux/2
  Integrator/1 -> Demux/1, Sum5/2
  Demux1/1 -> Product/2
  Compare To Constant/1 -> unsafeFlag/1
  Sum2/1 -> eh/1
  lcFlag/1 -> Switch/2
  xl/1 -> Sum/2
  Product/1 -> Sum7/1
  h/1 -> Mux/1
  Sum3/1 -> Sum2/2  "desired  gap"
  Sum1/1 -> Sum/1  "x (front bumber)"
  vf/1 -> Sum4/1, Product/1, Multiply/1
  Sum5/1 -> hFilterGain/1
  Switch/1 -> Sum5/1
  Demux/2 -> Sum3/2
  vLen/1 -> Sum1/1
  hLc/1 -> Mux1/1
  Demux1/2 -> Sum7/2
  Multiply/1 -> Sum3/1
  Sum/1 -> Sum6/1, "gap "/1, Sum2/1  "gap"
  xf/1 -> Sum1/2
  Demux/1 -> Multiply/2
  hFilterGain/1 -> Integrator/1
  d0Lc/1 -> Mux1/2
  Sum4/1 -> ev/1

== system full_maneuver_platoon_new_strategy/Lo/Vehicle Following During LC/Subsystem ==
  note: Condition for Gap Generating Vehicle
  note: Condition for Lane Changing Vehicle
  ego : Inport  OutDataTypeStr=Bus: vehStatesBus
  futureLeader : Inport  Port=2  OutDataTypeStr=Bus: vehStatesBus
  lcFlag : Inport  Port=3
  AND : Logic  IconShape=distinctive  AllPortsSameDT=off  OutDataTypeStr=boolean
  AND1 : Logic  IconShape=distinctive  AllPortsSameDT=off  OutDataTypeStr=boolean
  Abs : Abs
  Abs1 : Abs
  Bus Selector1 : BusSelector  OutputSignals=Y
  Bus Selector2 : BusSelector  OutputSignals=Y
  Compare To Constant : simulink/Logic and Bit Operations/Compare To Constant  relop=<=  const=1.8  OutDataTypeStr=boolean
  Compare To Constant1 : simulink/Logic and Bit Operations/Compare To Constant  relop=<=  const=0.5  OutDataTypeStr=boolean
  NOT : Logic  Operator=NOT  IconShape=distinctive  AllPortsSameDT=off  OutDataTypeStr=boolean
  OR : Logic  Operator=OR  IconShape=distinctive  AllPortsSameDT=off  OutDataTypeStr=boolean
  Scope : Scope  NumInputPorts=2
  Sum : Sum  Inputs=|+-
  Sum1 : Sum  Inputs=-+|
  lcDone : Outport
  wires:
  Abs1/1 -> Compare To Constant/1
  Abs/1 -> Compare To Constant1/1
  Bus Selector2/1 -> Sum1/2, Sum/1  "<Y>"
  AND1/1 -> OR/2, Scope/2
  OR/1 -> lcDone/1
  Compare To Constant1/1 -> AND1/2
  Sum1/1 -> Abs/1
  NOT/1 -> AND/2
  ego/1 -> Bus Selector2/1
  lcFlag/1 -> NOT/1, AND1/1
  Compare To Constant/1 -> AND/1
  Sum/1 -> Abs1/1
  AND/1 -> OR/1, Scope/1
  Bus Selector1/1 -> Sum/2, Sum1/1  "<Y>"
  futureLeader/1 -> Bus Selector1/1

== system full_maneuver_platoon_new_strategy/Lo/Vehicle Following During LC/Veh Following ==
  eh : Inport
  ev : Inport  Port=2
  realInput : Inport  Port=3
  intReset : Inport  Port=4
  Anti-windup gain : Gain  Gain=sqrt(Ki/Kd)
  Integrator : Integrator  ExternalReset=rising
  Kd : Gain  Gain=Kd
  Ki : Gain  Gain=Ki
  Kp : Gain  Gain=Kp
  Saturation1 : Saturate  UpperLimit=maxHeadwayError  LowerLimit=minHeadwayError
  Scope : Scope  NumInputPorts=4
  Sum : Sum  Inputs=|-+
  Sum1 : Sum  Inputs=+++
  Sum5 : Sum  Inputs=-+|
  u : Outport
  wires:
  ev/1 -> Kd/1
  Ki/1 -> Sum5/2
  Anti-windup gain/1 -> Sum5/1
  Sum5/1 -> Integrator/1
  Integrator/1 -> Sum1/1, Scope/1
  Kp/1 -> Sum1/2, Scope/2
  Kd/1 -> Scope/3, Sum1/3
  Saturation1/1 -> Kp/1, Ki/1
  eh/1 -> Saturation1/1
  Sum1/1 -> Sum/2, u/1, Scope/4
  realInput/1 -> Sum/1
  Sum/1 -> Anti-windup gain/1
  intReset/1 -> Integrator/2

== system full_maneuver_platoon_new_strategy/Lo/Vehicle Following During LC/Velocity Control ==
  velocity : Inport
  realInput : Inport  Port=2
  intReset : Inport  Port=3
  Anti-windup gain : Gain  Gain=velKp/velKi
  Integrator2 : Integrator  ExternalReset=falling
  Sum : Sum  Inputs=|+-
  Sum1 : Sum  Inputs=|-+
  Sum2 : Sum  Inputs=-+|
  Sum3 : Sum  Inputs=|++
  freeFlowVel : Constant  Value=freeFlowVel
  velKi : Gain  Gain=velKi
  velKp : Gain  Gain=velKp
  u : Outport
  wires:
  Sum/1 -> velKi/1, velKp/1
  velKp/1 -> Sum3/2
  velKi/1 -> Sum2/2
  Integrator2/1 -> Sum3/1
  velocity/1 -> Sum/2
  freeFlowVel/1 -> Sum/1
  intReset/1 -> Integrator2/2
  Sum3/1 -> Sum1/2, u/1
  Anti-windup gain/1 -> Sum2/1
  realInput/1 -> Sum1/1
  Sum1/1 -> Anti-windup gain/1
  Sum2/1 -> Integrator2/1

== system full_maneuver_platoon_new_strategy/Lo/Virtual Vehicle Following/Compute Errors ==
  xf : Inport
  vf : Inport  Port=2
  xl : Inport  Port=3
  vl : Inport  Port=4
  lcFlag : Inport  Port=5
  Compare To Constant : simulink/Logic and Bit Operations/Compare To Constant  relop=<=  const=0  OutDataTypeStr=boolean
  Demux : Demux  Outputs=2
  Demux1 : Demux  Outputs=2
  Gain3 : Gain  Gain=velFilterGain/10
  Integrator : Integrator  InitialCondition=[h d0]
  Integrator1 : Integrator  InitialCondition=vx0
  Multiply : Product
  Mux : Mux  Inputs=2
  Mux1 : Mux  Inputs=2
  Product : Product
  Saturation : Saturate  UpperLimit=maxAcceleration  LowerLimit=minAcceleration
  Sum : Sum  Inputs=-+|
  Sum1 : Sum  Inputs=++|
  Sum2 : Sum  Inputs=+-|
  Sum3 : Sum  Inputs=|++
  Sum4 : Sum  Inputs=-+|
  Sum5 : Sum  Inputs=|+-
  Sum6 : Sum  Inputs=+-|
  Sum7 : Sum  Inputs=|++
  Sum8 : Sum  Inputs=|+-
  Switch : Switch  Criteria=u2 > Threshold
  d0 : Constant  Value=d0
  d0Lc : Constant  Value=d0Lc
  h : Constant  Value=h
  hFilterGain : Gain  Gain=hFilterGain
  hLc : Constant  Value=hLc
  vLen : Constant  Value=lr+lf
  eh : Outport
  ev : Outport  Port=2
  "gap " : Outport  Port=3
  unsafeFlag : Outport  Port=4
  wires:
  vl/1 -> Sum8/1
  Saturation/1 -> Integrator1/1
  Sum8/1 -> Gain3/1
  Gain3/1 -> Saturation/1
  Integrator1/1 -> Sum8/2, Sum4/2
  Sum4/1 -> ev/1
  d0Lc/1 -> Mux1/2
  hFilterGain/1 -> Integrator/1
  Demux/1 -> Multiply/2
  xf/1 -> Sum1/2
  Sum/1 -> Sum2/1, "gap "/1, Sum6/1  "gap"
  Multiply/1 -> Sum3/1
  Demux1/2 -> Sum7/2
  hLc/1 -> Mux1/1
  vLen/1 -> Sum1/1
  Demux/2 -> Sum3/2
  Switch/1 -> Sum5/1
  Sum5/1 -> hFilterGain/1
  vf/1 -> Multiply/1, Product/1, Sum4/1
  Sum1/1 -> Sum/1  "x (front bumber)"
  Sum3/1 -> Sum2/2  "desired  gap"
  h/1 -> Mux/1
  Product/1 -> Sum7/1
  xl/1 -> Sum/2
  lcFlag/1 -> Switch/2
  Sum2/1 -> eh/1
  Compare To Constant/1 -> unsafeFlag/1
  Demux1/1 -> Product/2
  Integrator/1 -> Sum5/2, Demux/1
  d0/1 -> Mux/2
  Mux1/1 -> Switch/1
  Sum7/1 -> Sum6/2  "safe  gap"
  Mux/1 -> Switch/3, Demux1/1  "min safe gap"
  Sum6/1 -> Compare To Constant/1

== system full_maneuver_platoon_new_strategy/Lo/Virtual Vehicle Following/Subsystem ==
  ego : Inport  OutDataTypeStr=Bus: vehStatesBus
  virtualLeader : Inport  Port=2  OutDataTypeStr=Bus: vehStatesBus
  Abs : Abs
  Bus Selector : BusSelector  OutputSignals=Y
  Bus Selector1 : BusSelector  OutputSignals=Y
  Compare To Constant : simulink/Logic and Bit Operations/Compare To Constant  relop=<  const=3.6-0.5  OutDataTypeStr=boolean
  Scope : Scope  NumInputPorts=3
  Sum : Sum  Inputs=+-
  lcStarted : Outport
  wires:
  Abs/1 -> Compare To Constant/1, Scope/3
  Sum/1 -> Abs/1
  Compare To Constant/1 -> lcStarted/1
  Bus Selector1/1 -> Scope/2, Sum/2  "<Y>"
  Bus Selector/1 -> Sum/1, Scope/1  "<Y>"
  virtualLeader/1 -> Bus Selector1/1
  ego/1 -> Bus Selector/1

== system full_maneuver_platoon_new_strategy/Lo/Virtual Vehicle Following/Velocity Control ==
  note: Velocity control
  intReset : Inport
  ev : Inport  Port=2
  Integrator2 : Integrator  ExternalReset=rising
  Sum3 : Sum
  velKi : Gain  Gain=velKi
  velKp : Gain  Gain=velKp
  Out1 : Outport
  wires:
  intReset/1 -> Integrator2/2
  ev/1 -> Integrator2/1, velKp/1
  velKp/1 -> Sum3/1
  Sum3/1 -> Out1/1
  velKi/1 -> Sum3/2
  Integrator2/1 -> velKi/1

== system full_maneuver_platoon_new_strategy/Lo/Virtual Vehicle Following/Virtual Leader Following ==
  eh : Inport
  ev : Inport  Port=2
  realInput : Inport  Port=3
  Anti-windup gain : Gain  Gain=sqrt(Ki/Kd)
  Integrator : Integrator
  Kd : Gain  Gain=Kd
  Ki : Gain  Gain=Ki
  Kp : Gain  Gain=Kp
  Saturation1 : Saturate  UpperLimit=maxHeadwayError  LowerLimit=minHeadwayError
  Scope : Scope  NumInputPorts=3
  Sum : Sum  Inputs=|-+
  Sum1 : Sum  Inputs=+++
  Sum5 : Sum  Inputs=-+|
  u : Outport
  wires:
  Sum/1 -> Anti-windup gain/1
  realInput/1 -> Sum/1
  Sum1/1 -> u/1, Sum/2
  eh/1 -> Saturation1/1
  Saturation1/1 -> Ki/1, Kp/1
  Kd/1 -> Sum1/3, Scope/3
  Kp/1 -> Sum1/2, Scope/2
  Integrator/1 -> Sum1/1, Scope/1
  Sum5/1 -> Integrator/1
  Anti-windup gain/1 -> Sum5/1
  Ki/1 -> Sum5/2
  ev/1 -> Kd/1

== system full_maneuver_platoon_new_strategy/Lo/followerErrors/gapToFollower ==
  xf : Inport
  vf : Inport  Port=2
  xl : Inport  Port=3
  Multiply : Product
  Sum : Sum  Inputs=-+|
  Sum1 : Sum  Inputs=++|
  Sum2 : Sum  Inputs=+-|
  Sum3 : Sum  Inputs=|++
  d0 : Constant  Value=d0
  h : Constant  Value=h
  vLen : Constant  Value=lr+lf
  eh : Outport
  "gap " : Outport  Port=2
  wires:
  d0/1 -> Sum3/2  "gap at  standstill"
  h/1 -> Multiply/2  "time headway"
  Sum2/1 -> eh/1
  xl/1 -> Sum/2
  Sum1/1 -> Sum/1  "x (front bumber)"
  vf/1 -> Multiply/1
  Sum3/1 -> Sum2/2  "desired  gap"
  xf/1 -> Sum1/2
  Sum/1 -> Sum2/1, "gap "/1  "gap"
  Multiply/1 -> Sum3/1
  vLen/1 -> Sum1/1

== system full_maneuver_platoon_new_strategy/p1/Lateral Control/Full State Observer ==
  note: xhat
  note: yhat
  measuredOutputs : Inport
  delta : Inport  Port=2
  Add1 : Sum  Inputs=|-+
  Gain : Gain  Gain=B  Multiplication=Matrix(K*u)
  Gain1 : Gain  Gain=C  Multiplication=Matrix(K*u)
  Gain2 : Gain  Gain=L  Multiplication=Matrix(K*u)
  Gain3 : Gain  Gain=A  Multiplication=Matrix(K*u)
  Integrator : Integrator  InitialCondition=[y0; 0; 0; 0]
  Signal Specification : SignalSpecification  Dimensions=[size(C,1) 1]
  Sum : Sum  Inputs=+++
  xhat : Outport
  wires:
  Add1/1 -> Signal Specification/1
  Integrator/1 -> xhat/1, Gain3/1, Gain1/1
  Gain1/1 -> Add1/1
  Sum/1 -> Integrator/1
  measuredOutputs/1 -> Add1/2
  delta/1 -> Gain/1
  Gain/1 -> Sum/3
  Gain3/1 -> Sum/2
  Signal Specification/1 -> Gain2/1
  Gain2/1 -> Sum/1

== system full_maneuver_platoon_new_strategy/p1/Lateral Control/Triggered Subsystem1 ==
  In1 : Inport
  Trigger : TriggerPort  VariantControl=Variant
  Out1 : Outport  InitialOutput=y0
  wires:
  In1/1 -> Out1/1

== system full_maneuver_platoon_new_strategy/p1/Regular Vehicle Following/Compute Errors ==
  xf : Inport
  vf : Inport  Port=2
  xl : Inport  Port=3
  vl : Inport  Port=4
  extraSpaceFlag : Inport  Port=5
  Compare To Constant : simulink/Logic and Bit Operations/Compare To Constant  relop=<  const=-0.1  OutDataTypeStr=boolean
  Demux : Demux  Outputs=2
  Demux1 : Demux  Outputs=2
  Gain3 : Gain  Gain=velFilterGain
  Integrator : Integrator  InitialCondition=[h d0]
  Integrator1 : Integrator  InitialCondition=vx0
  Multiply : Product
  Mux : Mux  Inputs=2
  Mux1 : Mux  Inputs=2
  Product : Product
  Saturation : Saturate  UpperLimit=maxAcceleration  LowerLimit=minAcceleration
  Sum : Sum  Inputs=-+|
  Sum1 : Sum  Inputs=++|
  Sum2 : Sum  Inputs=+-|
  Sum3 : Sum  Inputs=|++
  Sum4 : Sum  Inputs=-+|
  Sum5 : Sum  Inputs=|+-
  Sum6 : Sum  Inputs=+-|
  Sum7 : Sum  Inputs=|++
  Sum8 : Sum  Inputs=|+-
  Switch : Switch  Criteria=u2 > Threshold
  d0 : Constant  Value=d0
  d0Lc : Constant  Value=d0Lc
  h : Constant  Value=h
  hFilterGain : Gain  Gain=hFilterGain
  hLc : Constant  Value=hLc
  vLen : Constant  Value=lr+lf
  eh : Outport
  ev : Outport  Port=2
  "gap " : Outport  Port=3
  unsafeFlag : Outport  Port=4
  wires:
  Sum8/1 -> Gain3/1
  Integrator1/1 -> Sum8/2, Sum4/2
  Saturation/1 -> Integrator1/1
  Gain3/1 -> Saturation/1
  Sum4/1 -> ev/1
  vl/1 -> Sum8/1
  d0Lc/1 -> Mux1/2
  hFilterGain/1 -> Integrator/1
  Demux/1 -> Multiply/2
  xf/1 -> Sum1/2
  Sum/1 -> Sum2/1, "gap "/1, Sum6/1  "gap"
  Multiply/1 -> Sum3/1
  Demux1/2 -> Sum7/2
  hLc/1 -> Mux1/1
  vLen/1 -> Sum1/1
  Demux/2 -> Sum3/2
  Switch/1 -> Sum5/1
  Sum5/1 -> hFilterGain/1
  vf/1 -> Multiply/1, Product/1, Sum4/1
  Sum1/1 -> Sum/1  "x (front bumber)"
  Sum3/1 -> Sum2/2  "desired  gap"
  h/1 -> Mux/1
  Product/1 -> Sum7/1
  xl/1 -> Sum/2
  extraSpaceFlag/1 -> Switch/2
  Sum2/1 -> eh/1
  Compare To Constant/1 -> unsafeFlag/1
  Demux1/1 -> Product/2
  Integrator/1 -> Sum5/2, Demux/1
  d0/1 -> Mux/2
  Mux1/1 -> Switch/1
  Sum7/1 -> Sum6/2  "safe  gap"
  Mux/1 -> Demux1/1, Switch/3  "min safe gap"
  Sum6/1 -> Compare To Constant/1

== system full_maneuver_platoon_new_strategy/p1/Regular Vehicle Following/Veh Following ==
  eh : Inport
  ev : Inport  Port=2
  realInput : Inport  Port=3
  intReset : Inport  Port=4
  Anti-windup gain : Gain  Gain=sqrt(Ki/Kd)
  Integrator : Integrator  ExternalReset=rising
  Kd : Gain  Gain=Kd
  Ki : Gain  Gain=Ki
  Kp : Gain  Gain=Kp
  Saturation1 : Saturate  UpperLimit=maxHeadwayError  LowerLimit=minHeadwayError
  Scope : Scope  NumInputPorts=4
  Sum : Sum  Inputs=|-+
  Sum1 : Sum  Inputs=+++
  Sum5 : Sum  Inputs=-+|
  u : Outport
  wires:
  intReset/1 -> Integrator/2
  Sum/1 -> Anti-windup gain/1
  realInput/1 -> Sum/1
  Sum1/1 -> Scope/4, u/1, Sum/2
  eh/1 -> Saturation1/1
  Saturation1/1 -> Ki/1, Kp/1
  Kd/1 -> Sum1/3, Scope/3
  Kp/1 -> Scope/2, Sum1/2
  Integrator/1 -> Scope/1, Sum1/1
  Sum5/1 -> Integrator/1
  Anti-windup gain/1 -> Sum5/1
  Ki/1 -> Sum5/2
  ev/1 -> Kd/1

== system full_maneuver_platoon_new_strategy/p1/Regular Vehicle Following/Velocity Control ==
  velocity : Inport
  realInput : Inport  Port=2
  intReset : Inport  Port=3
  Anti-windup gain : Gain  Gain=velKp/velKi
  Integrator2 : Integrator  ExternalReset=falling
  Sum : Sum  Inputs=|+-
  Sum1 : Sum  Inputs=|-+
  Sum2 : Sum  Inputs=-+|
  Sum3 : Sum  Inputs=|++
  freeFlowVel : Constant  Value=freeFlowVel
  velKi : Gain  Gain=velKi
  velKp : Gain  Gain=velKp
  u : Outport
  wires:
  Sum2/1 -> Integrator2/1
  Sum1/1 -> Anti-windup gain/1
  realInput/1 -> Sum1/1
  Anti-windup gain/1 -> Sum2/1
  Sum3/1 -> u/1, Sum1/2
  intReset/1 -> Integrator2/2
  freeFlowVel/1 -> Sum/1
  velocity/1 -> Sum/2
  Integrator2/1 -> Sum3/1
  velKi/1 -> Sum2/2
  velKp/1 -> Sum3/2
  Sum/1 -> velKp/1, velKi/1

== system full_maneuver_platoon_new_strategy/p1/Vehicle Following During LC/Compute Errors ==
  xf : Inport
  vf : Inport  Port=2
  xl : Inport  Port=3
  vl : Inport  Port=4
  extraSpaceFlag : Inport  Port=5
  Compare To Constant : simulink/Logic and Bit Operations/Compare To Constant  relop=<=  const=0  OutDataTypeStr=boolean
  Demux : Demux  Outputs=2
  Demux1 : Demux  Outputs=2
  Gain3 : Gain  Gain=velFilterGain
  Integrator : Integrator  InitialCondition=[h d0]
  Integrator1 : Integrator  InitialCondition=vx0
  Multiply : Product
  Mux : Mux  Inputs=2
  Mux1 : Mux  Inputs=2
  Product : Product
  Saturation : Saturate  UpperLimit=maxAcceleration  LowerLimit=minAcceleration
  Sum : Sum  Inputs=-+|
  Sum1 : Sum  Inputs=++|
  Sum2 : Sum  Inputs=+-|
  Sum3 : Sum  Inputs=|++
  Sum4 : Sum  Inputs=-+|
  Sum5 : Sum  Inputs=|+-
  Sum6 : Sum  Inputs=+-|
  Sum7 : Sum  Inputs=|++
  Sum8 : Sum  Inputs=|+-
  Switch : Switch  Criteria=u2 > Threshold
  d0 : Constant  Value=d0
  d0Lc : Constant  Value=d0Lc
  h : Constant  Value=h
  hFilterGain : Gain  Gain=hFilterGain
  hLc : Constant  Value=hLc
  vLen : Constant  Value=lr+lf
  eh : Outport
  ev : Outport  Port=2
  "gap " : Outport  Port=3
  unsafeFlag : Outport  Port=4
  wires:
  vl/1 -> Sum8/1
  Sum8/1 -> Gain3/1
  Integrator1/1 -> Sum8/2, Sum4/2
  Gain3/1 -> Saturation/1
  Saturation/1 -> Integrator1/1
  Sum6/1 -> Compare To Constant/1
  Mux/1 -> Demux1/1, Switch/3  "min safe gap"
  Sum7/1 -> Sum6/2  "safe  gap"
  Mux1/1 -> Switch/1
  d0/1 -> Mux/2
  Integrator/1 -> Demux/1, Sum5/2
  Demux1/1 -> Product/2
  Compare To Constant/1 -> unsafeFlag/1
  Sum2/1 -> eh/1
  extraSpaceFlag/1 -> Switch/2
  xl/1 -> Sum/2
  Product/1 -> Sum7/1
  h/1 -> Mux/1
  Sum3/1 -> Sum2/2  "desired  gap"
  Sum1/1 -> Sum/1  "x (front bumber)"
  vf/1 -> Sum4/1, Product/1, Multiply/1
  Sum5/1 -> hFilterGain/1
  Switch/1 -> Sum5/1
  Demux/2 -> Sum3/2
  vLen/1 -> Sum1/1
  hLc/1 -> Mux1/1
  Demux1/2 -> Sum7/2
  Multiply/1 -> Sum3/1
  Sum/1 -> Sum6/1, "gap "/1, Sum2/1  "gap"
  xf/1 -> Sum1/2
  Demux/1 -> Multiply/2
  hFilterGain/1 -> Integrator/1
  d0Lc/1 -> Mux1/2
  Sum4/1 -> ev/1

== system full_maneuver_platoon_new_strategy/p1/Vehicle Following During LC/Veh Following ==
  eh : Inport
  ev : Inport  Port=2
  realInput : Inport  Port=3
  intReset : Inport  Port=4
  Anti-windup gain : Gain  Gain=sqrt(Ki/Kd)
  Integrator : Integrator  ExternalReset=rising
  Kd : Gain  Gain=Kd
  Ki : Gain  Gain=Ki
  Kp : Gain  Gain=Kp
  Saturation1 : Saturate  UpperLimit=maxHeadwayError  LowerLimit=minHeadwayError
  Scope : Scope  NumInputPorts=4
  Sum : Sum  Inputs=|-+
  Sum1 : Sum  Inputs=+++
  Sum5 : Sum  Inputs=-+|
  u : Outport
  wires:
  ev/1 -> Kd/1
  Ki/1 -> Sum5/2
  Anti-windup gain/1 -> Sum5/1
  Sum5/1 -> Integrator/1
  Integrator/1 -> Sum1/1, Scope/1
  Kp/1 -> Sum1/2, Scope/2
  Kd/1 -> Scope/3, Sum1/3
  Saturation1/1 -> Kp/1, Ki/1
  eh/1 -> Saturation1/1
  Sum1/1 -> Sum/2, u/1, Scope/4
  realInput/1 -> Sum/1
  Sum/1 -> Anti-windup gain/1
  intReset/1 -> Integrator/2
